simulink model "LQR_test"  (R2023a)
settings: Solver=VariableStepAuto  StartTime=0.0  StopTime=1.5  MaxStep=1e-2  RelTol=1e-3
values from neighbouring files (symbols this model uses):
  A = [0    1    0   0 ... (first row only)    [parameter.m]    (also in ref.m = pa.A)
  B = [0; (I+m*l^2)/den; 0; -m*l/den]    [parameter.m]
undefined symbols (not defined in the file or in its folder): K
settings Model: Creator=edzel  LastModifiedBy=edzel

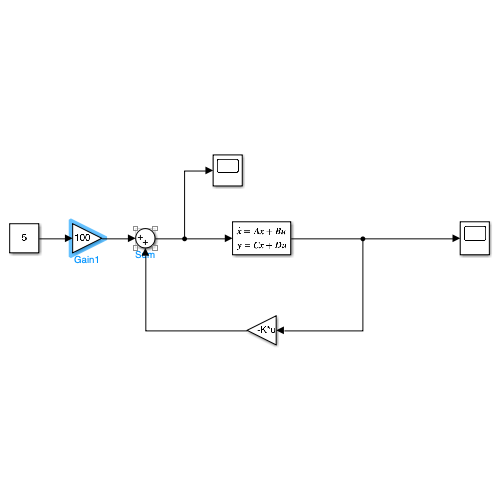
[thumbnail: Simulink's stored preview of the top-level diagram]
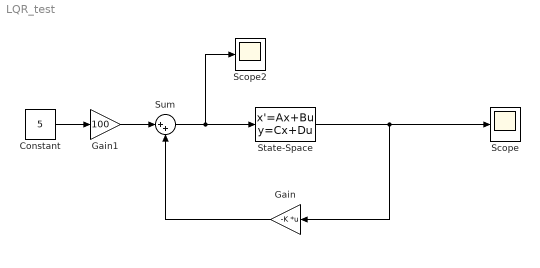
== system LQR_test ==
  Constant : Constant  Value=5
  Gain : Gain  Gain=-K  Multiplication=Matrix(K*u)
  Gain1 : Gain  Gain=100
  Scope : Scope
  Scope2 : Scope
  State-Space : StateSpace  A=A  B=B  C=eye(2)  D=[0; 0]  InitialCondition=0
  Sum : Sum  Inputs=|++
  wires:
  State-Space/1 -> Gain/1, Scope/1
  Gain/1 -> Sum/2
  Sum/1 -> Scope2/1, State-Space/1
  Constant/1 -> Gain1/1
  Gain1/1 -> Sum/1
